simulink model "preLookupTestGen21"  (R2017b)
settings: Solver=FixedStepDiscrete  StartTime=0.0  StopTime=10.0  RelTol=1e-3
undefined symbols (not defined in the file): Block_TestLib, enable
settings Model: Creator=ktrinh  LastModifiedBy=ktrinh
settings DebuggingCC: ParameterOverflowMsg=none

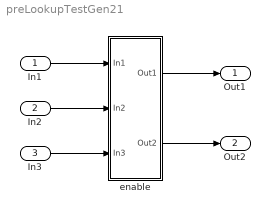
== system preLookupTestGen21 ==
  In1 : Inport
  In2 : Inport  Port=2
  In3 : Inport  Port=3
  enable : Subsystem  AncestorBlock=Block_TestLib/enable
  Out1 : Outport
  Out2 : Outport  Port=2
  wires:
  In1/1 -> enable/1(In1)
  In2/1 -> enable/2(In2)
  In3/1 -> enable/3(In3)
  enable/1(Out1) -> Out1/1
  enable/2(Out2) -> Out2/1

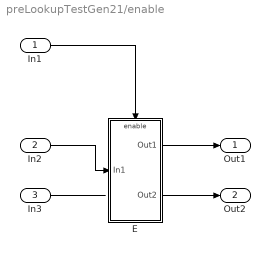
== system preLookupTestGen21/enable ==
  In1 : Inport  OutDataTypeStr=boolean
  In2 : Inport  Port=2
  In3 : Inport  Port=3
  E : Subsystem  TreatAsAtomicUnit=on
  Out1 : Outport
  Out2 : Outport  Port=2
  wires:
  In1/1 -> E/Enable
  In2/1 -> E/1(In1)
  In3/1 -> ?
  E/1(Out1) -> Out1/1
  E/2(Out2) -> Out2/1

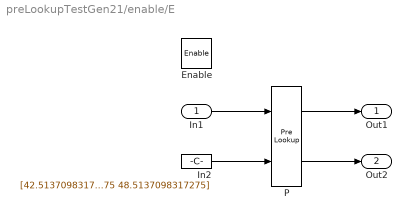
== system preLookupTestGen21/enable/E ==
  In1 : Inport  PortDimensions=1
  Enable : EnablePort
  In2 : Constant  Value=[42.5137098317275 44.0137098317275 45.5137098317275 47.0137098317275 48.5137098317275]
  P : PreLookup  BreakpointsDataSource=Input port  BreakpointsData=[10:10:110]  IndexSearchMethod=Linear search  ExtrapMethod=Linear  UseLastBreakpoint=on  BreakpointDataTypeStr=Inherit: Inherit from 'Breakpoint data'  IndexDataTypeStr=uint16  FractionDataTypeStr=single  RndMeth=Ceiling
      settings: InputPortMap=u0,p1
  Out1 : Outport
  Out2 : Outport  Port=2
  wires:
  In1/1 -> P/1
  In2/1 -> P/2
  P/1 -> Out1/1
  P/2 -> Out2/1
